simulink model "IEEE14_case"  (R2024b)
settings: Solver=FixedStepAuto  StartTime=0  StopTime=2  FixedStep=1e-7  RelTol=1e-3
values from neighbouring files (symbols this model uses):
  GFL_15_Bva = 0.009    [IEEE14_parameters.m]
  GFL_15_C_bus_pu = 7.179419    [IEEE14_parameters.m]
  GFL_15_f0 = 60    [IEEE14_parameters.m]
  GFL_15_I_id = 691.26967    [IEEE14_parameters.m]
  GFL_15_I_iq = 691.26967    [IEEE14_parameters.m]
  GFL_15_I_od = 45.2207    [IEEE14_parameters.m]
  GFL_15_I_oq = 45.2207    [IEEE14_parameters.m]
  GFL_15_I_pll = 0.78    [IEEE14_parameters.m]
  GFL_15_Kdi = 0.09    [IEEE14_parameters.m]
  GFL_15_Kdo = 0.9    [IEEE14_parameters.m]
  GFL_15_Kqi = 0.09    [IEEE14_parameters.m]
  GFL_15_Kqo = 0.9    [IEEE14_parameters.m]
  GFL_15_Lg_pu = 0.631447    [IEEE14_parameters.m]
  GFL_15_mode = 1    [IEEE14_parameters.m]
  GFL_15_P_id = 3.7166    [IEEE14_parameters.m]
  GFL_15_P_iq = 3.7166    [IEEE14_parameters.m]
  GFL_15_P_od = 0.4798    [IEEE14_parameters.m]
  GFL_15_P_oq = 0.4798    [IEEE14_parameters.m]
  GFL_15_P_pll = 290.42    [IEEE14_parameters.m]
  GFL_15_Qe_ref = 0.2    [IEEE14_parameters.m]
  GFL_15_Rg_pu = 0.024016    [IEEE14_parameters.m]
  GFL_15_Sbase = 1.000000e+4    (= 10000)    [IEEE14_parameters.m]
  GFL_15_Tdi = 0.01    [IEEE14_parameters.m]
  GFL_15_Tdo = 0.2    [IEEE14_parameters.m]
  GFL_15_Tqi = 0.01    [IEEE14_parameters.m]
  GFL_15_Tqo = 0.2    [IEEE14_parameters.m]
  GFL_15_Vbase = 380    [IEEE14_parameters.m]
  GFL_15_Vdc_ref = 1.011475    [IEEE14_parameters.m]
  GFL_15_Vdcbase = 700    [IEEE14_parameters.m]
  GFL_15_vq_ref = 0    [IEEE14_parameters.m]
  GFL_16_Bva = 0.002    [IEEE14_parameters.m]
  GFL_16_C_bus_pu = 7.179419    [IEEE14_parameters.m]
  GFL_16_f0 = 60    [IEEE14_parameters.m]
  GFL_16_I_id = 691.26967    [IEEE14_parameters.m]
  GFL_16_I_iq = 691.26967    [IEEE14_parameters.m]
  GFL_16_I_od = 45.2207    [IEEE14_parameters.m]
  GFL_16_I_oq = 45.2207    [IEEE14_parameters.m]
  GFL_16_I_pll = 0.78    [IEEE14_parameters.m]
  GFL_16_Kdi = 0.05    [IEEE14_parameters.m]
  GFL_16_Kdo = 0.5    [IEEE14_parameters.m]
  GFL_16_Kqi = 0.05    [IEEE14_parameters.m]
  GFL_16_Kqo = 0.5    [IEEE14_parameters.m]
  GFL_16_Lg_pu = 0.631447    [IEEE14_parameters.m]
  GFL_16_mode = 1    [IEEE14_parameters.m]
  GFL_16_P_id = 3.7166    [IEEE14_parameters.m]
  GFL_16_P_iq = 3.7166    [IEEE14_parameters.m]
  GFL_16_P_od = 0.4798    [IEEE14_parameters.m]
  GFL_16_P_oq = 0.4798    [IEEE14_parameters.m]
  GFL_16_P_pll = 290.42    [IEEE14_parameters.m]
  GFL_16_Qe_ref = 0.2    [IEEE14_parameters.m]
  GFL_16_Rg_pu = 0.024016    [IEEE14_parameters.m]
  GFL_16_Sbase = 1.000000e+4    (= 10000)    [IEEE14_parameters.m]
  GFL_16_Tdi = 0.01    [IEEE14_parameters.m]
  GFL_16_Tdo = 0.2    [IEEE14_parameters.m]
  GFL_16_Tqi = 0.01    [IEEE14_parameters.m]
  GFL_16_Tqo = 0.2    [IEEE14_parameters.m]
  GFL_16_Vbase = 380    [IEEE14_parameters.m]
  GFL_16_Vdc_ref = 1.01144    [IEEE14_parameters.m]
  GFL_16_Vdcbase = 700    [IEEE14_parameters.m]
  GFL_16_vq_ref = 0    [IEEE14_parameters.m]
  GFL_17_Bva = 0.002    [IEEE14_parameters.m]
  GFL_17_C_bus_pu = 7.179419    [IEEE14_parameters.m]
  GFL_17_f0 = 60    [IEEE14_parameters.m]
  GFL_17_I_id = 691.26967    [IEEE14_parameters.m]
  GFL_17_I_iq = 691.26967    [IEEE14_parameters.m]
  GFL_17_I_od = 45.2207    [IEEE14_parameters.m]
  GFL_17_I_oq = 45.2207    [IEEE14_parameters.m]
  GFL_17_I_pll = 0.78    [IEEE14_parameters.m]
  GFL_17_Kdi = 0.05    [IEEE14_parameters.m]
  GFL_17_Kdo = 0.5    [IEEE14_parameters.m]
  GFL_17_Kqi = 0.05    [IEEE14_parameters.m]
  GFL_17_Kqo = 0.5    [IEEE14_parameters.m]
  GFL_17_Lg_pu = 0.631447    [IEEE14_parameters.m]
  GFL_17_mode = 1    [IEEE14_parameters.m]
  GFL_17_P_id = 3.7166    [IEEE14_parameters.m]
  GFL_17_P_iq = 3.7166    [IEEE14_parameters.m]
  GFL_17_P_od = 0.4798    [IEEE14_parameters.m]
  GFL_17_P_oq = 0.4798    [IEEE14_parameters.m]
  GFL_17_P_pll = 290.42    [IEEE14_parameters.m]
  GFL_17_Qe_ref = 0.2    [IEEE14_parameters.m]
  GFL_17_Rg_pu = 0.024016    [IEEE14_parameters.m]
  GFL_17_Sbase = 1.000000e+4    (= 10000)    [IEEE14_parameters.m]
  GFL_17_Tdi = 0.01    [IEEE14_parameters.m]
  GFL_17_Tdo = 0.2    [IEEE14_parameters.m]
  GFL_17_Tqi = 0.01    [IEEE14_parameters.m]
  GFL_17_Tqo = 0.2    [IEEE14_parameters.m]
  GFL_17_Vbase = 380    [IEEE14_parameters.m]
  GFL_17_Vdc_ref = 1.011632    [IEEE14_parameters.m]
  GFL_17_Vdcbase = 700    [IEEE14_parameters.m]
  GFL_17_vq_ref = 0    [IEEE14_parameters.m]
  GFL_18_Bva = 0.002    [IEEE14_parameters.m]
  GFL_18_C_bus_pu = 7.179419    [IEEE14_parameters.m]
  GFL_18_f0 = 60    [IEEE14_parameters.m]
  GFL_18_I_id = 691.26967    [IEEE14_parameters.m]
  GFL_18_I_iq = 691.26967    [IEEE14_parameters.m]
  GFL_18_I_od = 45.2207    [IEEE14_parameters.m]
  GFL_18_I_oq = 45.2207    [IEEE14_parameters.m]
  GFL_18_I_pll = 0.78    [IEEE14_parameters.m]
  GFL_18_Kdi = 0.05    [IEEE14_parameters.m]
  GFL_18_Kdo = 0.5    [IEEE14_parameters.m]
  GFL_18_Kqi = 0.05    [IEEE14_parameters.m]
  GFL_18_Kqo = 0.5    [IEEE14_parameters.m]
  GFL_18_Lg_pu = 0.631447    [IEEE14_parameters.m]
  GFL_18_mode = 1    [IEEE14_parameters.m]
  GFL_18_P_id = 3.7166    [IEEE14_parameters.m]
  GFL_18_P_iq = 3.7166    [IEEE14_parameters.m]
  GFL_18_P_od = 0.4798    [IEEE14_parameters.m]
  GFL_18_P_oq = 0.4798    [IEEE14_parameters.m]
  GFL_18_P_pll = 290.42    [IEEE14_parameters.m]
  GFL_18_Qe_ref = 0.2    [IEEE14_parameters.m]
  GFL_18_Rg_pu = 0.024016    [IEEE14_parameters.m]
  GFL_18_Sbase = 1.000000e+4    (= 10000)    [IEEE14_parameters.m]
  GFL_18_Tdi = 0.01    [IEEE14_parameters.m]
  GFL_18_Tdo = 0.2    [IEEE14_parameters.m]
  GFL_18_Tqi = 0.01    [IEEE14_parameters.m]
  GFL_18_Tqo = 0.2    [IEEE14_parameters.m]
  GFL_18_Vbase = 380    [IEEE14_parameters.m]
  GFL_18_Vdc_ref = 1.011572    [IEEE14_parameters.m]
  GFL_18_Vdcbase = 700    [IEEE14_parameters.m]
  GFL_18_vq_ref = 0    [IEEE14_parameters.m]
  ... (+180 more)
(part 7 of 25)

== system IEEE14_case/AC_1/d_iq_line_4_9_block ==
  note: d_iq_line_4_9 in case14gfl
      | $699.506853548825\,\mathrm{vq}_{\mathrm{bus},4}-376.991118430775\,\mathrm{id}_{\mathrm{line},4,9}-699.506853548825\,\mathrm{vq}_{\mathrm{bus},9}$
      | Automatically generated on 2025-10-09 21:39:28 .
  State_id_line_4_9_5fb10 : Inport
  State_vq_bus_4_2d444 : Inport  Port=2
  State_vq_bus_9_e7de0 : Inport  Port=3
  Add_39299 : Sum
  Constant_-376.991118430775_3ea59 : Constant  Value=-376.991118430775
  Constant_699.506853548825_37d82 : Constant  Value=699.506853548825
  Constant_699.506853548825_6575b : Constant  Value=699.506853548825
  Product_2ea70 : Product
  Product_57b01 : Product
  Product_cf664 : Product
  Subtract_80e4f : Sum  Inputs=+-
  Blockout_d_iq_line_4_9_8879d : Outport
  wires:
  Constant_-376.991118430775_3ea59/1 -> Product_57b01/1
  Product_cf664/1 -> Add_39299/2
  Product_57b01/1 -> Add_39299/1
  State_id_line_4_9_5fb10/1 -> Product_57b01/2
  Constant_699.506853548825_6575b/1 -> Product_cf664/1
  State_vq_bus_4_2d444/1 -> Product_cf664/2
  Product_2ea70/1 -> Subtract_80e4f/2
  Constant_699.506853548825_37d82/1 -> Product_2ea70/1
  State_vq_bus_9_e7de0/1 -> Product_2ea70/2
  Add_39299/1 -> Subtract_80e4f/1
  Subtract_80e4f/1 -> Blockout_d_iq_line_4_9_8879d/1

== system IEEE14_case/AC_1/d_iq_line_5_6_block ==
  note: d_iq_line_5_6 in case14gfl
      | $1605.01907859506\,\mathrm{vq}_{\mathrm{bus},5}-376.991118430775\,\mathrm{id}_{\mathrm{line},5,6}-1605.01907859506\,\mathrm{vq}_{\mathrm{bus},6}$
      | Automatically generated on 2025-10-09 21:39:30 .
  State_id_line_5_6_8d92b : Inport
  State_vq_bus_5_491c0 : Inport  Port=2
  State_vq_bus_6_39104 : Inport  Port=3
  Add_7c3b3 : Sum
  Constant_-376.991118430775_fdd64 : Constant  Value=-376.991118430775
  Constant_1605.01907859506_0c9f5 : Constant  Value=1605.01907859506
  Constant_1605.01907859506_7f4c8 : Constant  Value=1605.01907859506
  Product_35d69 : Product
  Product_b6bdb : Product
  Product_ff1a8 : Product
  Subtract_873d9 : Sum  Inputs=+-
  Blockout_d_iq_line_5_6_9d95c : Outport
  wires:
  Constant_-376.991118430775_fdd64/1 -> Product_ff1a8/1
  Product_ff1a8/1 -> Add_7c3b3/1
  State_id_line_5_6_8d92b/1 -> Product_ff1a8/2
  Constant_1605.01907859506_0c9f5/1 -> Product_35d69/1
  State_vq_bus_5_491c0/1 -> Product_35d69/2
  Product_35d69/1 -> Add_7c3b3/2
  State_vq_bus_6_39104/1 -> Product_b6bdb/2
  Product_b6bdb/1 -> Subtract_873d9/2
  Constant_1605.01907859506_7f4c8/1 -> Product_b6bdb/1
  Add_7c3b3/1 -> Subtract_873d9/1
  Subtract_873d9/1 -> Blockout_d_iq_line_5_6_9d95c/1

== system IEEE14_case/AC_1/d_iq_line_6_11_block ==
  note: d_iq_line_6_11 in case14gfl
      | $1895.38018316126\,\mathrm{vq}_{\mathrm{bus},6}-180.023209796657\,\mathrm{iq}_{\mathrm{line},6,11}-376.991118430775\,\mathrm{id}_{\mathrm{line},6,11}-1895.38018316126\,\mathrm{vq}_{\mathrm{bus},11}$
      | Automatically generated on 2025-10-09 21:39:32 .
  State_id_line_6_11_3e498 : Inport
  State_iq_line_6_11_23688 : Inport  Port=2
  State_vq_bus_11_5a0e6 : Inport  Port=3
  State_vq_bus_6_fa1ab : Inport  Port=4
  Add_f0066 : Sum
  Constant_-376.991118430775_7fe8b : Constant  Value=-376.991118430775
  Constant_180.023209796657_42678 : Constant  Value=180.023209796657
  Constant_1895.38018316126_7900e : Constant  Value=1895.38018316126
  Constant_1895.38018316126_a1828 : Constant  Value=1895.38018316126
  Product_3a14e : Product
  Product_60b79 : Product
  Product_843e4 : Product
  Product_bb537 : Product
  Subtract_7b150 : Sum  Inputs=+-
  Subtract_c1d87 : Sum  Inputs=+-
  Blockout_d_iq_line_6_11_ea354 : Outport
  wires:
  Product_60b79/1 -> Subtract_7b150/1
  Constant_-376.991118430775_7fe8b/1 -> Product_60b79/1
  State_id_line_6_11_3e498/1 -> Product_60b79/2
  Constant_180.023209796657_42678/1 -> Product_3a14e/1
  Product_3a14e/1 -> Subtract_7b150/2
  State_iq_line_6_11_23688/1 -> Product_3a14e/2
  Product_bb537/1 -> Subtract_c1d87/2
  Subtract_7b150/1 -> Subtract_c1d87/1
  Constant_1895.38018316126_a1828/1 -> Product_bb537/1
  State_vq_bus_11_5a0e6/1 -> Product_bb537/2
  Product_843e4/1 -> Add_f0066/2
  Constant_1895.38018316126_7900e/1 -> Product_843e4/1
  State_vq_bus_6_fa1ab/1 -> Product_843e4/2
  Subtract_c1d87/1 -> Add_f0066/1
  Add_f0066/1 -> Blockout_d_iq_line_6_11_ea354/1

== system IEEE14_case/AC_1/d_iq_line_6_12_block ==
  note: d_iq_line_6_12 in case14gfl
      | $1473.7153294663\,\mathrm{vq}_{\mathrm{bus},6}-181.134351144703\,\mathrm{iq}_{\mathrm{line},6,12}-376.991118430775\,\mathrm{id}_{\mathrm{line},6,12}-1473.7153294663\,\mathrm{vq}_{\mathrm{bus},12}$
      | Automatically generated on 2025-10-09 21:39:34 .
  State_id_line_6_12_268a8 : Inport
  State_iq_line_6_12_950d7 : Inport  Port=2
  State_vq_bus_12_69550 : Inport  Port=3
  State_vq_bus_6_e763a : Inport  Port=4
  Add_b7468 : Sum
  Constant_-376.991118430775_f1d4f : Constant  Value=-376.991118430775
  Constant_1473.7153294663_049d6 : Constant  Value=1473.7153294663
  Constant_1473.7153294663_ac463 : Constant  Value=1473.7153294663
  Constant_181.134351144703_38039 : Constant  Value=181.134351144703
  Product_43b5c : Product
  Product_574f5 : Product
  Product_5ec2e : Product
  Product_93b39 : Product
  Subtract_6d476 : Sum  Inputs=+-
  Subtract_ac6c5 : Sum  Inputs=+-
  Blockout_d_iq_line_6_12_bda61 : Outport
  wires:
  Subtract_ac6c5/1 -> Subtract_6d476/1
  Constant_-376.991118430775_f1d4f/1 -> Product_574f5/1
  Product_574f5/1 -> Subtract_ac6c5/1
  State_id_line_6_12_268a8/1 -> Product_574f5/2
  Constant_181.134351144703_38039/1 -> Product_43b5c/1
  Product_43b5c/1 -> Subtract_ac6c5/2
  Product_93b39/1 -> Subtract_6d476/2
  Constant_1473.7153294663_049d6/1 -> Product_93b39/1
  State_iq_line_6_12_950d7/1 -> Product_43b5c/2
  State_vq_bus_12_69550/1 -> Product_93b39/2
  Constant_1473.7153294663_ac463/1 -> Product_5ec2e/1
  State_vq_bus_6_e763a/1 -> Product_5ec2e/2
  Subtract_6d476/1 -> Add_b7468/1
  Product_5ec2e/1 -> Add_b7468/2
  Add_b7468/1 -> Blockout_d_iq_line_6_12_bda61/1

== system IEEE14_case/AC_1/d_iq_line_6_13_block ==
  note: d_iq_line_6_13 in case14gfl
      | $2893.92122845456\,\mathrm{vq}_{\mathrm{bus},6}-191.432889262269\,\mathrm{iq}_{\mathrm{line},6,13}-376.991118430775\,\mathrm{id}_{\mathrm{line},6,13}-2893.92122845456\,\mathrm{vq}_{\mathrm{bus},13}$
      | Automatically generated on 2025-10-09 21:39:36 .
  State_id_line_6_13_f1d85 : Inport
  State_iq_line_6_13_f7b4b : Inport  Port=2
  State_vq_bus_13_5730a : Inport  Port=3
  State_vq_bus_6_f0e31 : Inport  Port=4
  Add_1c903 : Sum
  Constant_-376.991118430775_5ef0e : Constant  Value=-376.991118430775
  Constant_191.432889262269_5c0fd : Constant  Value=191.432889262269
  Constant_2893.92122845456_a0aba : Constant  Value=2893.92122845456
  Constant_2893.92122845456_a4a61 : Constant  Value=2893.92122845456
  Product_0336c : Product
  Product_1b8db : Product
  Product_302cd : Product
  Product_77864 : Product
  Subtract_80e31 : Sum  Inputs=+-
  Subtract_b1026 : Sum  Inputs=+-
  Blockout_d_iq_line_6_13_6bd96 : Outport
  wires:
  Constant_-376.991118430775_5ef0e/1 -> Product_0336c/1
  Constant_191.432889262269_5c0fd/1 -> Product_1b8db/1
  State_id_line_6_13_f1d85/1 -> Product_0336c/2
  Product_1b8db/1 -> Subtract_b1026/2
  State_iq_line_6_13_f7b4b/1 -> Product_1b8db/2
  Product_77864/1 -> Subtract_80e31/2
  Constant_2893.92122845456_a0aba/1 -> Product_77864/1
  Product_0336c/1 -> Subtract_b1026/1
  State_vq_bus_13_5730a/1 -> Product_77864/2
  Subtract_b1026/1 -> Subtract_80e31/1
  Product_302cd/1 -> Add_1c903/2
  Constant_2893.92122845456_a4a61/1 -> Product_302cd/1
  State_vq_bus_6_f0e31/1 -> Product_302cd/2
  Subtract_80e31/1 -> Add_1c903/1
  Add_1c903/1 -> Blockout_d_iq_line_6_13_6bd96/1

== system IEEE14_case/AC_1/d_iq_line_7_8_block ==
  note: d_iq_line_7_8 in case14gfl
      | $2140.17098172453\,\mathrm{vq}_{\mathrm{bus},7}-376.991118430775\,\mathrm{id}_{\mathrm{line},7,8}-2140.17098172453\,\mathrm{vq}_{\mathrm{bus},8}$
      | Automatically generated on 2025-10-09 21:39:38 .
  State_id_line_7_8_32461 : Inport
  State_vq_bus_7_4632e : Inport  Port=2
  State_vq_bus_8_957c7 : Inport  Port=3
  Add_fd8d6 : Sum
  Constant_-376.991118430775_d615e : Constant  Value=-376.991118430775
  Constant_2140.17098172453_9f9e4 : Constant  Value=2140.17098172453
  Constant_2140.17098172453_c3816 : Constant  Value=2140.17098172453
  Product_142e7 : Product
  Product_f2e78 : Product
  Product_f7504 : Product
  Subtract_6e91e : Sum  Inputs=+-
  Blockout_d_iq_line_7_8_a0a04 : Outport
  wires:
  Constant_-376.991118430775_d615e/1 -> Product_f2e78/1
  Product_f2e78/1 -> Add_fd8d6/1
  State_id_line_7_8_32461/1 -> Product_f2e78/2
  Constant_2140.17098172453_c3816/1 -> Product_142e7/1
  Product_142e7/1 -> Add_fd8d6/2
  Product_f7504/1 -> Subtract_6e91e/2
  Constant_2140.17098172453_9f9e4/1 -> Product_f7504/1
  State_vq_bus_7_4632e/1 -> Product_142e7/2
  State_vq_bus_8_957c7/1 -> Product_f7504/2
  Add_fd8d6/1 -> Subtract_6e91e/1
  Subtract_6e91e/1 -> Blockout_d_iq_line_7_8_a0a04/1

== system IEEE14_case/AC_1/d_iq_line_7_9_block ==
  note: d_iq_line_7_9 in case14gfl
      | $3426.88045114785\,\mathrm{vq}_{\mathrm{bus},7}-376.991118430775\,\mathrm{id}_{\mathrm{line},7,9}-3426.88045114785\,\mathrm{vq}_{\mathrm{bus},9}$
      | Automatically generated on 2025-10-09 21:39:40 .
  State_id_line_7_9_a5037 : Inport
  State_vq_bus_7_de92f : Inport  Port=2
  State_vq_bus_9_3c7a5 : Inport  Port=3
  Add_30ef7 : Sum
  Constant_-376.991118430775_e9a53 : Constant  Value=-376.991118430775
  Constant_3426.88045114785_151c5 : Constant  Value=3426.88045114785
  Constant_3426.88045114785_ad75e : Constant  Value=3426.88045114785
  Product_648d8 : Product
  Product_dc9ab : Product
  Product_e3dd0 : Product
  Subtract_73145 : Sum  Inputs=+-
  Blockout_d_iq_line_7_9_01bdc : Outport
  wires:
  State_vq_bus_9_3c7a5/1 -> Product_dc9ab/2
  Constant_-376.991118430775_e9a53/1 -> Product_e3dd0/1
  Product_dc9ab/1 -> Subtract_73145/2
  Product_e3dd0/1 -> Add_30ef7/1
  Constant_3426.88045114785_151c5/1 -> Product_dc9ab/1
  State_id_line_7_9_a5037/1 -> Product_e3dd0/2
  Constant_3426.88045114785_ad75e/1 -> Product_648d8/1
  State_vq_bus_7_de92f/1 -> Product_648d8/2
  Product_648d8/1 -> Add_30ef7/2
  Add_30ef7/1 -> Subtract_73145/1
  Subtract_73145/1 -> Blockout_d_iq_line_7_9_01bdc/1

== system IEEE14_case/AC_1/d_iq_line_9_10_block ==
  note: d_iq_line_9_10 in case14gfl
      | $4461.43335421036\,\mathrm{vq}_{\mathrm{bus},9}-141.918194997431\,\mathrm{iq}_{\mathrm{line},9,10}-376.991118430775\,\mathrm{id}_{\mathrm{line},9,10}-4461.43335421036\,\mathrm{vq}_{\mathrm{bus},10}$
      | Automatically generated on 2025-10-09 21:39:42 .
  State_id_line_9_10_7d192 : Inport
  State_iq_line_9_10_78cd2 : Inport  Port=2
  State_vq_bus_10_aebb4 : Inport  Port=3
  State_vq_bus_9_d6463 : Inport  Port=4
  Add_9c341 : Sum
  Constant_-376.991118430775_01110 : Constant  Value=-376.991118430775
  Constant_141.918194997431_f967c : Constant  Value=141.918194997431
  Constant_4461.43335421036_69f6f : Constant  Value=4461.43335421036
  Constant_4461.43335421036_9672c : Constant  Value=4461.43335421036
  Product_02b9f : Product
  Product_1253c : Product
  Product_45f04 : Product
  Product_d2758 : Product
  Subtract_137d4 : Sum  Inputs=+-
  Subtract_6b3b6 : Sum  Inputs=+-
  Blockout_d_iq_line_9_10_9f0b6 : Outport
  wires:
  Constant_-376.991118430775_01110/1 -> Product_1253c/1
  Add_9c341/1 -> Blockout_d_iq_line_9_10_9f0b6/1
  State_id_line_9_10_7d192/1 -> Product_1253c/2
  Constant_141.918194997431_f967c/1 -> Product_45f04/1
  Product_45f04/1 -> Subtract_137d4/2
  State_vq_bus_10_aebb4/1 -> Product_02b9f/2
  State_iq_line_9_10_78cd2/1 -> Product_45f04/2
  Product_1253c/1 -> Subtract_137d4/1
  Constant_4461.43335421036_69f6f/1 -> Product_02b9f/1
  Subtract_137d4/1 -> Subtract_6b3b6/1
  Product_02b9f/1 -> Subtract_6b3b6/2
  Product_d2758/1 -> Add_9c341/2
  Constant_4461.43335421036_9672c/1 -> Product_d2758/1
  State_vq_bus_9_d6463/1 -> Product_d2758/2
  Subtract_6b3b6/1 -> Add_9c341/1

== system IEEE14_case/AC_1/d_iq_line_9_14_block ==
  note: d_iq_line_9_14 in case14gfl
      | $1394.30105196677\,\mathrm{vq}_{\mathrm{bus},9}-177.229606715496\,\mathrm{iq}_{\mathrm{line},9,14}-376.991118430775\,\mathrm{id}_{\mathrm{line},9,14}-1394.30105196677\,\mathrm{vq}_{\mathrm{bus},14}$
      | Automatically generated on 2025-10-09 21:39:45 .
  State_id_line_9_14_dd4a4 : Inport
  State_iq_line_9_14_07292 : Inport  Port=2
  State_vq_bus_14_753fc : Inport  Port=3
  State_vq_bus_9_d4758 : Inport  Port=4
  Add_8f103 : Sum
  Constant_-376.991118430775_6bc62 : Constant  Value=-376.991118430775
  Constant_1394.30105196677_50c0c : Constant  Value=1394.30105196677
  Constant_1394.30105196677_acb93 : Constant  Value=1394.30105196677
  Constant_177.229606715496_1731d : Constant  Value=177.229606715496
  Product_21531 : Product
  Product_30771 : Product
  Product_33e78 : Product
  Product_cf39f : Product
  Subtract_51c64 : Sum  Inputs=+-
  Subtract_b0fd6 : Sum  Inputs=+-
  Blockout_d_iq_line_9_14_f1895 : Outport
  wires:
  Constant_-376.991118430775_6bc62/1 -> Product_21531/1
  State_id_line_9_14_dd4a4/1 -> Product_21531/2
  Subtract_b0fd6/1 -> Subtract_51c64/1
  Constant_177.229606715496_1731d/1 -> Product_30771/1
  Product_30771/1 -> Subtract_b0fd6/2
  Product_cf39f/1 -> Subtract_51c64/2
  Constant_1394.30105196677_50c0c/1 -> Product_cf39f/1
  State_iq_line_9_14_07292/1 -> Product_30771/2
  Product_21531/1 -> Subtract_b0fd6/1
  State_vq_bus_14_753fc/1 -> Product_cf39f/2
  Product_33e78/1 -> Add_8f103/2
  Constant_1394.30105196677_acb93/1 -> Product_33e78/1
  State_vq_bus_9_d4758/1 -> Product_33e78/2
  Subtract_51c64/1 -> Add_8f103/1
  Add_8f103/1 -> Blockout_d_iq_line_9_14_f1895/1

== system IEEE14_case/AC_1/d_iq_load_10_block ==
  note: d_iq_load_10 in case14gfl
      | $60.6278129379132\,\mathrm{vq}_{\mathrm{bus},10}-584.986218254651\,\mathrm{iq}_{\mathrm{load},10}-376.991118430775\,\mathrm{id}_{\mathrm{load},10}$
      | Automatically generated on 2025-10-09 21:39:02 .
  State_id_load_10_0a094 : Inport
  State_iq_load_10_0f9f7 : Inport  Port=2
  State_vq_bus_10_81f02 : Inport  Port=3
  Add_d132c : Sum
  Constant_-376.991118430775_0f5ea : Constant  Value=-376.991118430775
  Constant_584.986218254651_56ed2 : Constant  Value=584.986218254651
  Constant_60.6278129379132_5da5b : Constant  Value=60.6278129379132
  Product_310ba : Product
  Product_360f0 : Product
  Product_4d8c0 : Product
  Subtract_ea92d : Sum  Inputs=+-
  Blockout_d_iq_load_10_8a684 : Outport
  wires:
  State_id_load_10_0a094/1 -> Product_4d8c0/2
  Constant_-376.991118430775_0f5ea/1 -> Product_4d8c0/1
  Constant_584.986218254651_56ed2/1 -> Product_360f0/1
  Product_360f0/1 -> Subtract_ea92d/2
  Product_310ba/1 -> Add_d132c/2
  Constant_60.6278129379132_5da5b/1 -> Product_310ba/1
  State_iq_load_10_0f9f7/1 -> Product_360f0/2
  Product_4d8c0/1 -> Subtract_ea92d/1
  State_vq_bus_10_81f02/1 -> Product_310ba/2
  Subtract_ea92d/1 -> Add_d132c/1
  Add_d132c/1 -> Blockout_d_iq_load_10_8a684/1

== system IEEE14_case/AC_1/d_iq_load_11_block ==
  note: d_iq_load_11 in case14gfl
      | $26.9582940185634\,\mathrm{vq}_{\mathrm{bus},11}-733.038285837618\,\mathrm{iq}_{\mathrm{load},11}-376.991118430775\,\mathrm{id}_{\mathrm{load},11}$
      | Automatically generated on 2025-10-09 21:39:04 .
  State_id_load_11_9ab2f : Inport
  State_iq_load_11_f52d6 : Inport  Port=2
  State_vq_bus_11_ff375 : Inport  Port=3
  Add_de68f : Sum
  Constant_-376.991118430775_db176 : Constant  Value=-376.991118430775
  Constant_26.9582940185634_925bd : Constant  Value=26.9582940185634
  Constant_733.038285837618_6ff3b : Constant  Value=733.038285837618
  Product_491fa : Product
  Product_5b80d : Product
  Product_c6838 : Product
  Subtract_79916 : Sum  Inputs=+-
  Blockout_d_iq_load_11_90745 : Outport
  wires:
  Constant_-376.991118430775_db176/1 -> Product_491fa/1
  Constant_733.038285837618_6ff3b/1 -> Product_c6838/1
  Product_c6838/1 -> Subtract_79916/2
  State_id_load_11_9ab2f/1 -> Product_491fa/2
  State_iq_load_11_f52d6/1 -> Product_c6838/2
  Product_491fa/1 -> Subtract_79916/1
  State_vq_bus_11_ff375/1 -> Product_5b80d/2
  Product_5b80d/1 -> Add_de68f/2
  Constant_26.9582940185634_925bd/1 -> Product_5b80d/1
  Subtract_79916/1 -> Add_de68f/1
  Add_de68f/1 -> Blockout_d_iq_load_11_90745/1

== system IEEE14_case/AC_1/d_iq_load_12_block ==
  note: d_iq_load_12 in case14gfl
      | $77.623450441014\,\mathrm{vq}_{\mathrm{bus},12}-1437.27863901733\,\mathrm{iq}_{\mathrm{load},12}-376.991118430775\,\mathrm{id}_{\mathrm{load},12}$
      | Automatically generated on 2025-10-09 21:39:06 .
  State_id_load_12_0975f : Inport
  State_iq_load_12_acbdc : Inport  Port=2
  State_vq_bus_12_83802 : Inport  Port=3
  Add_36107 : Sum
  Constant_-376.991118430775_9dcd8 : Constant  Value=-376.991118430775
  Constant_1437.27863901733_57e09 : Constant  Value=1437.27863901733
  Constant_77.623450441014_2708c : Constant  Value=77.623450441014
  Product_a0656 : Product
  Product_c6599 : Product
  Product_e67ca : Product
  Subtract_88912 : Sum  Inputs=+-
  Blockout_d_iq_load_12_9f109 : Outport
  wires:
  State_id_load_12_0975f/1 -> Product_c6599/2
  Constant_-376.991118430775_9dcd8/1 -> Product_c6599/1
  Constant_1437.27863901733_57e09/1 -> Product_e67ca/1
  Product_e67ca/1 -> Subtract_88912/2
  Product_a0656/1 -> Add_36107/2
  Constant_77.623450441014_2708c/1 -> Product_a0656/1
  State_iq_load_12_acbdc/1 -> Product_e67ca/2
  Product_c6599/1 -> Subtract_88912/1
  State_vq_bus_12_83802/1 -> Product_a0656/2
  Subtract_88912/1 -> Add_36107/1
  Add_36107/1 -> Blockout_d_iq_load_12_9f109/1

== system IEEE14_case/AC_1/d_iq_load_13_block ==
  note: d_iq_load_13 in case14gfl
      | $118.242352238424\,\mathrm{vq}_{\mathrm{bus},13}-877.479327381977\,\mathrm{iq}_{\mathrm{load},13}-376.991118430775\,\mathrm{id}_{\mathrm{load},13}$
      | Automatically generated on 2025-10-09 21:39:07 .
  State_id_load_13_29b8c : Inport
  State_iq_load_13_dc329 : Inport  Port=2
  State_vq_bus_13_7eda7 : Inport  Port=3
  Add_196d0 : Sum
  Constant_-376.991118430775_54985 : Constant  Value=-376.991118430775
  Constant_118.242352238424_0be43 : Constant  Value=118.242352238424
  Constant_877.479327381977_663e1 : Constant  Value=877.479327381977
  Product_31344 : Product
  Product_8bd14 : Product
  Product_fe9c5 : Product
  Subtract_4cd3e : Sum  Inputs=+-
  Blockout_d_iq_load_13_714c3 : Outport
  wires:
  Constant_-376.991118430775_54985/1 -> Product_8bd14/1
  Constant_877.479327381977_663e1/1 -> Product_fe9c5/1
  Product_fe9c5/1 -> Subtract_4cd3e/2
  State_id_load_13_29b8c/1 -> Product_8bd14/2
  State_iq_load_13_dc329/1 -> Product_fe9c5/2
  Product_8bd14/1 -> Subtract_4cd3e/1
  State_vq_bus_13_7eda7/1 -> Product_31344/2
  Product_31344/1 -> Add_196d0/2
  Constant_118.242352238424_0be43/1 -> Product_31344/1
  Subtract_4cd3e/1 -> Add_196d0/1
  Add_196d0/1 -> Blockout_d_iq_load_13_714c3/1

== system IEEE14_case/AC_1/d_iq_load_14_block ==
  note: d_iq_load_14 in case14gfl
      | $156.099712947555\,\mathrm{vq}_{\mathrm{bus},14}-1123.43353292371\,\mathrm{iq}_{\mathrm{load},14}-376.991118430775\,\mathrm{id}_{\mathrm{load},14}$
      | Automatically generated on 2025-10-09 21:39:10 .
  State_id_load_14_07147 : Inport
  State_iq_load_14_ef373 : Inport  Port=2
  State_vq_bus_14_cd634 : Inport  Port=3
  Add_ad506 : Sum
  Constant_-376.991118430775_2060a : Constant  Value=-376.991118430775
  Constant_1123.43353292371_be503 : Constant  Value=1123.43353292371
  Constant_156.099712947555_a0693 : Constant  Value=156.099712947555
  Product_1a567 : Product
  Product_350ab : Product
  Product_37ef4 : Product
  Subtract_77877 : Sum  Inputs=+-
  Blockout_d_iq_load_14_aff57 : Outport
  wires:
  Constant_-376.991118430775_2060a/1 -> Product_350ab/1
  State_id_load_14_07147/1 -> Product_350ab/2
  Constant_1123.43353292371_be503/1 -> Product_1a567/1
  Product_1a567/1 -> Subtract_77877/2
  State_iq_load_14_ef373/1 -> Product_1a567/2
  Product_350ab/1 -> Subtract_77877/1
  State_vq_bus_14_cd634/1 -> Product_37ef4/2
  Add_ad506/1 -> Blockout_d_iq_load_14_aff57/1
  Product_37ef4/1 -> Add_ad506/2
  Constant_156.099712947555_a0693/1 -> Product_37ef4/1
  Subtract_77877/1 -> Add_ad506/1

== system IEEE14_case/AC_1/d_iq_load_2_block ==
  note: d_iq_load_2 in case14gfl
      | $171.84447318187\,\mathrm{vq}_{\mathrm{bus},2}-644.150178736049\,\mathrm{iq}_{\mathrm{load},2}-376.991118430775\,\mathrm{id}_{\mathrm{load},2}$
      | Automatically generated on 2025-10-09 21:38:51 .
  State_id_load_2_e4c0e : Inport
  State_iq_load_2_39818 : Inport  Port=2
  State_vq_bus_2_25b3a : Inport  Port=3
  Add_3d549 : Sum
  Constant_-376.991118430775_94e96 : Constant  Value=-376.991118430775
  Constant_171.84447318187_7b304 : Constant  Value=171.84447318187
  Constant_644.150178736049_dd5b8 : Constant  Value=644.150178736049
  Product_4ba83 : Product
  Product_91cb5 : Product
  Product_b6ea5 : Product
  Subtract_dfcdb : Sum  Inputs=+-
  Blockout_d_iq_load_2_9dea5 : Outport
  wires:
  Constant_-376.991118430775_94e96/1 -> Product_4ba83/1
  State_id_load_2_e4c0e/1 -> Product_4ba83/2
  Constant_644.150178736049_dd5b8/1 -> Product_b6ea5/1
  Product_b6ea5/1 -> Subtract_dfcdb/2
  State_iq_load_2_39818/1 -> Product_b6ea5/2
  Product_4ba83/1 -> Subtract_dfcdb/1
  State_vq_bus_2_25b3a/1 -> Product_91cb5/2
  Product_91cb5/1 -> Add_3d549/2
  Constant_171.84447318187_7b304/1 -> Product_91cb5/1
  Subtract_dfcdb/1 -> Add_3d549/1
  Add_3d549/1 -> Blockout_d_iq_load_2_9dea5/1

== system IEEE14_case/AC_1/d_iq_load_3_block ==
  note: d_iq_load_3 in case14gfl
      | $1796.20019807427\,\mathrm{vq}_{\mathrm{bus},3}-1869.08228190416\,\mathrm{iq}_{\mathrm{load},3}-376.991118430775\,\mathrm{id}_{\mathrm{load},3}$
      | Automatically generated on 2025-10-09 21:38:53 .
  State_id_load_3_d79a9 : Inport
  State_iq_load_3_276a1 : Inport  Port=2
  State_vq_bus_3_60dd0 : Inport  Port=3
  Add_0c614 : Sum
  Constant_-376.991118430775_2482b : Constant  Value=-376.991118430775
  Constant_1796.20019807427_a8905 : Constant  Value=1796.20019807427
  Constant_1869.08228190416_d8dae : Constant  Value=1869.08228190416
  Product_0f39e : Product
  Product_a564c : Product
  Product_a7995 : Product
  Subtract_ed118 : Sum  Inputs=+-
  Blockout_d_iq_load_3_49ef1 : Outport
  wires:
  Constant_-376.991118430775_2482b/1 -> Product_a564c/1
  State_id_load_3_d79a9/1 -> Product_a564c/2
  Constant_1869.08228190416_d8dae/1 -> Product_0f39e/1
  Product_0f39e/1 -> Subtract_ed118/2
  Product_a7995/1 -> Add_0c614/2
  Constant_1796.20019807427_a8905/1 -> Product_a7995/1
  State_iq_load_3_276a1/1 -> Product_0f39e/2
  Product_a564c/1 -> Subtract_ed118/1
  State_vq_bus_3_60dd0/1 -> Product_a7995/2
  Subtract_ed118/1 -> Add_0c614/1
  Add_0c614/1 -> Blockout_d_iq_load_3_49ef1/1

== system IEEE14_case/AC_1/d_iq_load_4_block ==
  note: d_iq_load_4 in case14gfl
      | $2007.66181460144\,\mathrm{vq}_{\mathrm{bus},4}-4620.55781051053\,\mathrm{iq}_{\mathrm{load},4}-376.991118430775\,\mathrm{id}_{\mathrm{load},4}$
      | Automatically generated on 2025-10-09 21:38:54 .
  State_id_load_4_3f12c : Inport
  State_iq_load_4_d8cb8 : Inport  Port=2
  State_vq_bus_4_a0870 : Inport  Port=3
  Add_0450e : Sum
  Constant_-376.991118430775_4db17 : Constant  Value=-376.991118430775
  Constant_2007.66181460144_721d3 : Constant  Value=2007.66181460144
  Constant_4620.55781051053_0d5fe : Constant  Value=4620.55781051053
  Product_5cc4f : Product
  Product_8d04b : Product
  Product_ee59e : Product
  Subtract_4e0cc : Sum  Inputs=+-
  Blockout_d_iq_load_4_a1a6f : Outport
  wires:
  Constant_-376.991118430775_4db17/1 -> Product_5cc4f/1
  Constant_4620.55781051053_0d5fe/1 -> Product_ee59e/1
  Product_ee59e/1 -> Subtract_4e0cc/2
  State_id_load_4_3f12c/1 -> Product_5cc4f/2
  State_iq_load_4_d8cb8/1 -> Product_ee59e/2
  Product_8d04b/1 -> Add_0450e/2
  Constant_2007.66181460144_721d3/1 -> Product_8d04b/1
  Product_5cc4f/1 -> Subtract_4e0cc/1
  State_vq_bus_4_a0870/1 -> Product_8d04b/2
  Subtract_4e0cc/1 -> Add_0450e/1
  Add_0450e/1 -> Blockout_d_iq_load_4_a1a6f/1

== system IEEE14_case/AC_1/d_iq_load_5_block ==
  note: d_iq_load_5 in case14gfl
      | $126.842875202809\,\mathrm{vq}_{\mathrm{bus},5}-1790.70781254618\,\mathrm{iq}_{\mathrm{load},5}-376.991118430775\,\mathrm{id}_{\mathrm{load},5}$
      | Automatically generated on 2025-10-09 21:38:56 .
  State_id_load_5_e43f2 : Inport
  State_iq_load_5_ed9b4 : Inport  Port=2
  State_vq_bus_5_cfb62 : Inport  Port=3
  Add_95bc5 : Sum
  Constant_-376.991118430775_cfec7 : Constant  Value=-376.991118430775
  Constant_126.842875202809_9c550 : Constant  Value=126.842875202809
  Constant_1790.70781254618_74583 : Constant  Value=1790.70781254618
  Product_15d6e : Product
  Product_20eec : Product
  Product_b8d9d : Product
  Subtract_fe7d7 : Sum  Inputs=+-
  Blockout_d_iq_load_5_ab2ba : Outport
  wires:
  State_id_load_5_e43f2/1 -> Product_20eec/2
  Constant_-376.991118430775_cfec7/1 -> Product_20eec/1
  Constant_1790.70781254618_74583/1 -> Product_15d6e/1
  Product_15d6e/1 -> Subtract_fe7d7/2
  State_iq_load_5_ed9b4/1 -> Product_15d6e/2
  Product_20eec/1 -> Subtract_fe7d7/1
  Product_b8d9d/1 -> Add_95bc5/2
  Constant_126.842875202809_9c550/1 -> Product_b8d9d/1
  State_vq_bus_5_cfb62/1 -> Product_b8d9d/2
  Subtract_fe7d7/1 -> Add_95bc5/1
  Add_95bc5/1 -> Blockout_d_iq_load_5_ab2ba/1

== system IEEE14_case/AC_1/d_iq_load_6_block ==
  note: d_iq_load_6 in case14gfl
      | $79.7688488749381\,\mathrm{vq}_{\mathrm{bus},6}-562.973403523291\,\mathrm{iq}_{\mathrm{load},6}-376.991118430775\,\mathrm{id}_{\mathrm{load},6}$
      | Automatically generated on 2025-10-09 21:38:58 .
  State_id_load_6_8bda4 : Inport
  State_iq_load_6_40498 : Inport  Port=2
  State_vq_bus_6_34215 : Inport  Port=3
  Add_60b3d : Sum
  Constant_-376.991118430775_c5b6b : Constant  Value=-376.991118430775
  Constant_562.973403523291_b5b01 : Constant  Value=562.973403523291
  Constant_79.7688488749381_4dbb0 : Constant  Value=79.7688488749381
  Product_ab997 : Product
  Product_aeba3 : Product
  Product_e7d90 : Product
  Subtract_99f0e : Sum  Inputs=+-
  Blockout_d_iq_load_6_d9bfd : Outport
  wires:
  Constant_-376.991118430775_c5b6b/1 -> Product_aeba3/1
  State_id_load_6_8bda4/1 -> Product_aeba3/2
  Constant_562.973403523291_b5b01/1 -> Product_e7d90/1
  Product_e7d90/1 -> Subtract_99f0e/2
  State_iq_load_6_40498/1 -> Product_e7d90/2
  Product_aeba3/1 -> Subtract_99f0e/1
  State_vq_bus_6_34215/1 -> Product_ab997/2
  Product_ab997/1 -> Add_60b3d/2
  Constant_79.7688488749381_4dbb0/1 -> Product_ab997/1
  Subtract_99f0e/1 -> Add_60b3d/1
  Add_60b3d/1 -> Blockout_d_iq_load_6_d9bfd/1

== system IEEE14_case/AC_1/d_iq_load_9_block ==
  note: d_iq_load_9 in case14gfl
      | $214.658794552347\,\mathrm{vq}_{\mathrm{bus},9}-669.954096006498\,\mathrm{iq}_{\mathrm{load},9}-376.991118430775\,\mathrm{id}_{\mathrm{load},9}$
      | Automatically generated on 2025-10-09 21:39:00 .
  State_id_load_9_c0f8a : Inport
  State_iq_load_9_3e6fb : Inport  Port=2
  State_vq_bus_9_1c480 : Inport  Port=3
  Add_e4dd6 : Sum
  Constant_-376.991118430775_e7f7f : Constant  Value=-376.991118430775
  Constant_214.658794552347_a4e84 : Constant  Value=214.658794552347
  Constant_669.954096006498_74fba : Constant  Value=669.954096006498
  Product_06427 : Product
  Product_4c7f8 : Product
  Product_84118 : Product
  Subtract_6bfbd : Sum  Inputs=+-
  Blockout_d_iq_load_9_c9e01 : Outport
  wires:
  Constant_-376.991118430775_e7f7f/1 -> Product_06427/1
  State_iq_load_9_3e6fb/1 -> Product_84118/2
  State_id_load_9_c0f8a/1 -> Product_06427/2
  Constant_669.954096006498_74fba/1 -> Product_84118/1
  Product_84118/1 -> Subtract_6bfbd/2
  Product_06427/1 -> Subtract_6bfbd/1
  State_vq_bus_9_1c480/1 -> Product_4c7f8/2
  Product_4c7f8/1 -> Add_e4dd6/2
  Constant_214.658794552347_a4e84/1 -> Product_4c7f8/1
  Subtract_6bfbd/1 -> Add_e4dd6/1
  Add_e4dd6/1 -> Blockout_d_iq_load_9_c9e01/1

== system IEEE14_case/AC_1/d_vd_bus_10_block ==
  note: d_vd_bus_10 in case14gfl
      | $1749.67102824962\,\mathrm{id}_{\mathrm{bus},10}+376.991118430775\,\mathrm{vq}_{\mathrm{bus},10}$
      | Automatically generated on 2025-10-09 21:38:36 .
  Alge_id_bus_10_8b36b : Inport
  State_vq_bus_10_6f6de : Inport  Port=2
  Add_a3e5f : Sum
  Constant_1749.67102824962_7c636 : Constant  Value=1749.67102824962
  Constant_376.991118430775_b349f : Constant  Value=376.991118430775
  Product_26821 : Product
  Product_27b5f : Product
  Blockout_d_vd_bus_10_484a7 : Outport
  wires:
  State_vq_bus_10_6f6de/1 -> Product_26821/2
  Constant_1749.67102824962_7c636/1 -> Product_27b5f/1
  Product_26821/1 -> Add_a3e5f/2
  Constant_376.991118430775_b349f/1 -> Product_26821/1
  Alge_id_bus_10_8b36b/1 -> Product_27b5f/2
  Product_27b5f/1 -> Add_a3e5f/1
  Add_a3e5f/1 -> Blockout_d_vd_bus_10_484a7/1

== system IEEE14_case/AC_1/d_vd_bus_11_block ==
  note: d_vd_bus_11 in case14gfl
      | $9002.98797417909\,\mathrm{id}_{\mathrm{bus},11}+376.991118430775\,\mathrm{vq}_{\mathrm{bus},11}$
      | Automatically generated on 2025-10-09 21:38:37 .
  Alge_id_bus_11_fad28 : Inport
  State_vq_bus_11_98fc3 : Inport  Port=2
  Add_c4251 : Sum
  Constant_376.991118430775_68760 : Constant  Value=376.991118430775
  Constant_9002.98797417909_f6ff4 : Constant  Value=9002.98797417909
  Product_61a89 : Product
  Product_8f0d7 : Product
  Blockout_d_vd_bus_11_0b5d5 : Outport
  wires:
  Alge_id_bus_11_fad28/1 -> Product_8f0d7/2
  Constant_9002.98797417909_f6ff4/1 -> Product_8f0d7/1
  Product_61a89/1 -> Add_c4251/2
  Constant_376.991118430775_68760/1 -> Product_61a89/1
  State_vq_bus_11_98fc3/1 -> Product_61a89/2
  Product_8f0d7/1 -> Add_c4251/1
  Add_c4251/1 -> Blockout_d_vd_bus_11_0b5d5/1

== system IEEE14_case/AC_1/d_vd_bus_12_block ==
  note: d_vd_bus_12 in case14gfl
      | $3672.44450708959\,\mathrm{id}_{\mathrm{bus},12}+376.991118430775\,\mathrm{vq}_{\mathrm{bus},12}$
      | Automatically generated on 2025-10-09 21:38:39 .
  Alge_id_bus_12_768d8 : Inport
  State_vq_bus_12_ee0ac : Inport  Port=2
  Add_1268c : Sum
  Constant_3672.44450708959_414e0 : Constant  Value=3672.44450708959
  Constant_376.991118430775_f9b2f : Constant  Value=376.991118430775
  Product_2ec96 : Product
  Product_d4bb7 : Product
  Blockout_d_vd_bus_12_63d51 : Outport
  wires:
  Add_1268c/1 -> Blockout_d_vd_bus_12_63d51/1
  Constant_3672.44450708959_414e0/1 -> Product_d4bb7/1
  Alge_id_bus_12_768d8/1 -> Product_d4bb7/2
  Constant_376.991118430775_f9b2f/1 -> Product_2ec96/1
  Product_d4bb7/1 -> Add_1268c/1
  State_vq_bus_12_ee0ac/1 -> Product_2ec96/2
  Product_2ec96/1 -> Add_1268c/2

== system IEEE14_case/AC_1/d_vd_bus_13_block ==
  note: d_vd_bus_13 in case14gfl
      | $2548.2341972351\,\mathrm{id}_{\mathrm{bus},13}+376.991118430775\,\mathrm{vq}_{\mathrm{bus},13}$
      | Automatically generated on 2025-10-09 21:38:40 .
  Alge_id_bus_13_3078a : Inport
  State_vq_bus_13_424b0 : Inport  Port=2
  Add_3ff77 : Sum
  Constant_2548.2341972351_a6f15 : Constant  Value=2548.2341972351
  Constant_376.991118430775_7edab : Constant  Value=376.991118430775
  Product_471d9 : Product
  Product_5ea4f : Product
  Blockout_d_vd_bus_13_9076d : Outport
  wires:
  Add_3ff77/1 -> Blockout_d_vd_bus_13_9076d/1
  Constant_2548.2341972351_a6f15/1 -> Product_5ea4f/1
  Alge_id_bus_13_3078a/1 -> Product_5ea4f/2
  Product_471d9/1 -> Add_3ff77/2
  Constant_376.991118430775_7edab/1 -> Product_471d9/1
  Product_5ea4f/1 -> Add_3ff77/1
  State_vq_bus_13_424b0/1 -> Product_471d9/2

== system IEEE14_case/AC_1/d_vd_bus_14_block ==
  note: d_vd_bus_14 in case14gfl
      | $20061.7254996805\,\mathrm{id}_{\mathrm{bus},14}+376.991118430775\,\mathrm{vq}_{\mathrm{bus},14}$
      | Automatically generated on 2025-10-09 21:38:42 .
  Alge_id_bus_14_7a3c0 : Inport
  State_vq_bus_14_3a1f7 : Inport  Port=2
  Add_09018 : Sum
  Constant_20061.7254996805_ad767 : Constant  Value=20061.7254996805
  Constant_376.991118430775_38c4b : Constant  Value=376.991118430775
  Product_0d21c : Product
  Product_9c99d : Product
  Blockout_d_vd_bus_14_7c236 : Outport
  wires:
  Constant_20061.7254996805_ad767/1 -> Product_9c99d/1
  Alge_id_bus_14_7a3c0/1 -> Product_9c99d/2
  Product_0d21c/1 -> Add_09018/2
  Constant_376.991118430775_38c4b/1 -> Product_0d21c/1
  Product_9c99d/1 -> Add_09018/1
  State_vq_bus_14_3a1f7/1 -> Product_0d21c/2
  Add_09018/1 -> Blockout_d_vd_bus_14_7c236/1

== system IEEE14_case/AC_1/d_vd_bus_15_block ==
  note: d_vd_bus_15 in case14gfl
      | $37699.1118430775\,\mathrm{id}_{\mathrm{bus},15}+376.991118430775\,\mathrm{vq}_{\mathrm{bus},15}$
      | Automatically generated on 2025-10-09 21:38:43 .
  Alge_id_bus_15_fd09e : Inport
  State_vq_bus_15_3aaea : Inport  Port=2
  Add_0b317 : Sum
  Constant_376.991118430775_00aaa : Constant  Value=376.991118430775
  Constant_37699.1118430775_a5440 : Constant  Value=37699.1118430775
  Product_cad66 : Product
  Product_d5012 : Product
  Blockout_d_vd_bus_15_6b2d1 : Outport
  wires:
  Constant_37699.1118430775_a5440/1 -> Product_cad66/1
  Product_d5012/1 -> Add_0b317/2
  Constant_376.991118430775_00aaa/1 -> Product_d5012/1
  Alge_id_bus_15_fd09e/1 -> Product_cad66/2
  State_vq_bus_15_3aaea/1 -> Product_d5012/2
  Product_cad66/1 -> Add_0b317/1
  Add_0b317/1 -> Blockout_d_vd_bus_15_6b2d1/1

== system IEEE14_case/AC_1/d_vd_bus_16_block ==
  note: d_vd_bus_16 in case14gfl
      | $37699.1118430775\,\mathrm{id}_{\mathrm{bus},16}+376.991118430775\,\mathrm{vq}_{\mathrm{bus},16}$
      | Automatically generated on 2025-10-09 21:38:45 .
  Alge_id_bus_16_8d52e : Inport
  State_vq_bus_16_21a55 : Inport  Port=2
  Add_c7ade : Sum
  Constant_376.991118430775_804af : Constant  Value=376.991118430775
  Constant_37699.1118430775_7bd68 : Constant  Value=37699.1118430775
  Product_435b3 : Product
  Product_53fa4 : Product
  Blockout_d_vd_bus_16_67f66 : Outport
  wires:
  Constant_37699.1118430775_7bd68/1 -> Product_435b3/1
  Product_53fa4/1 -> Add_c7ade/2
  Alge_id_bus_16_8d52e/1 -> Product_435b3/2
  Constant_376.991118430775_804af/1 -> Product_53fa4/1
  State_vq_bus_16_21a55/1 -> Product_53fa4/2
  Product_435b3/1 -> Add_c7ade/1
  Add_c7ade/1 -> Blockout_d_vd_bus_16_67f66/1

== system IEEE14_case/AC_1/d_vd_bus_17_block ==
  note: d_vd_bus_17 in case14gfl
      | $37699.1118430775\,\mathrm{id}_{\mathrm{bus},17}+376.991118430775\,\mathrm{vq}_{\mathrm{bus},17}$
      | Automatically generated on 2025-10-09 21:38:47 .
  Alge_id_bus_17_262b4 : Inport
  State_vq_bus_17_647a1 : Inport  Port=2
  Add_3de89 : Sum
  Constant_376.991118430775_c8c2f : Constant  Value=376.991118430775
  Constant_37699.1118430775_bffe4 : Constant  Value=37699.1118430775
  Product_5c0d6 : Product
  Product_68ad7 : Product
  Blockout_d_vd_bus_17_dc311 : Outport
  wires:
  Add_3de89/1 -> Blockout_d_vd_bus_17_dc311/1
  Constant_37699.1118430775_bffe4/1 -> Product_68ad7/1
  Alge_id_bus_17_262b4/1 -> Product_68ad7/2
  Product_5c0d6/1 -> Add_3de89/2
  Constant_376.991118430775_c8c2f/1 -> Product_5c0d6/1
  Product_68ad7/1 -> Add_3de89/1
  State_vq_bus_17_647a1/1 -> Product_5c0d6/2

== system IEEE14_case/AC_1/d_vd_bus_18_block ==
  note: d_vd_bus_18 in case14gfl
      | $37699.1118430775\,\mathrm{id}_{\mathrm{bus},18}+376.991118430775\,\mathrm{vq}_{\mathrm{bus},18}$
      | Automatically generated on 2025-10-09 21:38:48 .
  Alge_id_bus_18_48e95 : Inport
  State_vq_bus_18_c75a6 : Inport  Port=2
  Add_27cba : Sum
  Constant_376.991118430775_127bc : Constant  Value=376.991118430775
  Constant_37699.1118430775_f9a28 : Constant  Value=37699.1118430775
  Product_322c1 : Product
  Product_5453a : Product
  Blockout_d_vd_bus_18_49967 : Outport
  wires:
  Constant_37699.1118430775_f9a28/1 -> Product_5453a/1
  Alge_id_bus_18_48e95/1 -> Product_5453a/2
  Product_322c1/1 -> Add_27cba/2
  Constant_376.991118430775_127bc/1 -> Product_322c1/1
  Product_5453a/1 -> Add_27cba/1
  State_vq_bus_18_c75a6/1 -> Product_322c1/2
  Add_27cba/1 -> Blockout_d_vd_bus_18_49967/1

== system IEEE14_case/AC_1/d_vd_bus_1_block ==
  note: d_vd_bus_1 in case14gfl
      | $7391.98271432892\,\mathrm{id}_{\mathrm{bus},1}+376.991118430775\,\mathrm{vq}_{\mathrm{bus},1}$
      | Automatically generated on 2025-10-09 21:38:23 .
  Alge_id_bus_1_90b3c : Inport
  State_vq_bus_1_8d526 : Inport  Port=2
  Add_1c0b8 : Sum
  Constant_376.991118430775_8c1e4 : Constant  Value=376.991118430775
  Constant_7391.98271432892_c2a8f : Constant  Value=7391.98271432892
  Product_57029 : Product
  Product_6660f : Product
  Blockout_d_vd_bus_1_52715 : Outport
  wires:
  Constant_7391.98271432892_c2a8f/1 -> Product_57029/1
  Alge_id_bus_1_90b3c/1 -> Product_57029/2
  Product_6660f/1 -> Add_1c0b8/2
  Constant_376.991118430775_8c1e4/1 -> Product_6660f/1
  State_vq_bus_1_8d526/1 -> Product_6660f/2
  Add_1c0b8/1 -> Blockout_d_vd_bus_1_52715/1
  Product_57029/1 -> Add_1c0b8/1

== system IEEE14_case/AC_1/d_vd_bus_2_block ==
  note: d_vd_bus_2 in case14gfl
      | $4564.05712385926\,\mathrm{id}_{\mathrm{bus},2}+376.991118430775\,\mathrm{vq}_{\mathrm{bus},2}$
      | Automatically generated on 2025-10-09 21:38:24 .
  Alge_id_bus_2_b20cd : Inport
  State_vq_bus_2_bcae6 : Inport  Port=2
  Add_71e21 : Sum
  Constant_376.991118430775_c9454 : Constant  Value=376.991118430775
  Constant_4564.05712385926_b3c45 : Constant  Value=4564.05712385926
  Product_65c83 : Product
  Product_7d359 : Product
  Blockout_d_vd_bus_2_7ca8e : Outport
  wires:
  Constant_4564.05712385926_b3c45/1 -> Product_65c83/1
  Alge_id_bus_2_b20cd/1 -> Product_65c83/2
  Product_7d359/1 -> Add_71e21/2
  Constant_376.991118430775_c9454/1 -> Product_7d359/1
  Product_65c83/1 -> Add_71e21/1
  State_vq_bus_2_bcae6/1 -> Product_7d359/2
  Add_71e21/1 -> Blockout_d_vd_bus_2_7ca8e/1

== system IEEE14_case/AC_1/d_vd_bus_3_block ==
  note: d_vd_bus_3 in case14gfl
      | $13321.2409339497\,\mathrm{id}_{\mathrm{bus},3}+376.991118430775\,\mathrm{vq}_{\mathrm{bus},3}$
      | Automatically generated on 2025-10-09 21:38:26 .
  Alge_id_bus_3_b82db : Inport
  State_vq_bus_3_fe7bf : Inport  Port=2
  Add_0338a : Sum
  Constant_13321.2409339497_512f8 : Constant  Value=13321.2409339497
  Constant_376.991118430775_f70c2 : Constant  Value=376.991118430775
  Product_92891 : Product
  Product_ee890 : Product
  Blockout_d_vd_bus_3_5883d : Outport
  wires:
  Add_0338a/1 -> Blockout_d_vd_bus_3_5883d/1
  Constant_13321.2409339497_512f8/1 -> Product_92891/1
  Alge_id_bus_3_b82db/1 -> Product_92891/2
  Product_ee890/1 -> Add_0338a/2
  Constant_376.991118430775_f70c2/1 -> Product_ee890/1
  Product_92891/1 -> Add_0338a/1
  State_vq_bus_3_fe7bf/1 -> Product_ee890/2

== system IEEE14_case/AC_1/d_vd_bus_4_block ==
  note: d_vd_bus_4 in case14gfl
      | $2583.02077551357\,\mathrm{id}_{\mathrm{bus},4}+376.991118430775\,\mathrm{vq}_{\mathrm{bus},4}$
      | Automatically generated on 2025-10-09 21:38:27 .
  Alge_id_bus_4_f94e7 : Inport
  State_vq_bus_4_a1d9b : Inport  Port=2
  Add_04297 : Sum
  Constant_2583.02077551357_562d1 : Constant  Value=2583.02077551357
  Constant_376.991118430775_25894 : Constant  Value=376.991118430775
  Product_bf91e : Product
  Product_eba07 : Product
  Blockout_d_vd_bus_4_c11bd : Outport
  wires:
  Constant_2583.02077551357_562d1/1 -> Product_bf91e/1
  Alge_id_bus_4_f94e7/1 -> Product_bf91e/2
  Constant_376.991118430775_25894/1 -> Product_eba07/1
  Product_eba07/1 -> Add_04297/2
  State_vq_bus_4_a1d9b/1 -> Product_eba07/2
  Product_bf91e/1 -> Add_04297/1
  Add_04297/1 -> Blockout_d_vd_bus_4_c11bd/1

== system IEEE14_case/AC_1/d_vd_bus_5_block ==
  note: d_vd_bus_5 in case14gfl
      | $1402.86696243716\,\mathrm{id}_{\mathrm{bus},5}+376.991118430775\,\mathrm{vq}_{\mathrm{bus},5}$
      | Automatically generated on 2025-10-09 21:38:29 .
  Alge_id_bus_5_3a39c : Inport
  State_vq_bus_5_bfac5 : Inport  Port=2
  Add_800e2 : Sum
  Constant_1402.86696243716_2fe9f : Constant  Value=1402.86696243716
  Constant_376.991118430775_3c04e : Constant  Value=376.991118430775
  Product_db852 : Product
  Product_fcb25 : Product
  Blockout_d_vd_bus_5_c33ea : Outport
  wires:
  Constant_1402.86696243716_2fe9f/1 -> Product_db852/1
  Product_fcb25/1 -> Add_800e2/2
  Constant_376.991118430775_3c04e/1 -> Product_fcb25/1
  Alge_id_bus_5_3a39c/1 -> Product_db852/2
  State_vq_bus_5_bfac5/1 -> Product_fcb25/2
  Product_db852/1 -> Add_800e2/1
  Add_800e2/1 -> Blockout_d_vd_bus_5_c33ea/1

== system IEEE14_case/AC_1/d_vd_bus_6_block ==
  note: d_vd_bus_6 in case14gfl
      | $1302.18631108196\,\mathrm{id}_{\mathrm{bus},6}+376.991118430775\,\mathrm{vq}_{\mathrm{bus},6}$
      | Automatically generated on 2025-10-09 21:38:30 .
  Alge_id_bus_6_e431e : Inport
  State_vq_bus_6_681db : Inport  Port=2
  Add_45f75 : Sum
  Constant_1302.18631108196_58a93 : Constant  Value=1302.18631108196
  Constant_376.991118430775_e434a : Constant  Value=376.991118430775
  Product_72558 : Product
  Product_d1184 : Product
  Blockout_d_vd_bus_6_b094f : Outport
  wires:
  Constant_1302.18631108196_58a93/1 -> Product_72558/1
  Alge_id_bus_6_e431e/1 -> Product_72558/2
  Product_d1184/1 -> Add_45f75/2
  Constant_376.991118430775_e434a/1 -> Product_d1184/1
  State_vq_bus_6_681db/1 -> Product_d1184/2
  Product_72558/1 -> Add_45f75/1
  Add_45f75/1 -> Blockout_d_vd_bus_6_b094f/1

== system IEEE14_case/AC_1/d_vd_bus_7_block ==
  note: d_vd_bus_7 in case14gfl
      | $3504.63555759756\,\mathrm{id}_{\mathrm{bus},7}+376.991118430775\,\mathrm{vq}_{\mathrm{bus},7}$
      | Automatically generated on 2025-10-09 21:38:31 .
  Alge_id_bus_7_a7561 : Inport
  State_vq_bus_7_3c6fe : Inport  Port=2
  Add_4dc3a : Sum
  Constant_3504.63555759756_8bb38 : Constant  Value=3504.63555759756
  Constant_376.991118430775_26820 : Constant  Value=376.991118430775
  Product_37962 : Product
  Product_40e3b : Product
  Blockout_d_vd_bus_7_1c15c : Outport
  wires:
  Add_4dc3a/1 -> Blockout_d_vd_bus_7_1c15c/1
  Constant_3504.63555759756_8bb38/1 -> Product_40e3b/1
  Alge_id_bus_7_a7561/1 -> Product_40e3b/2
  Product_37962/1 -> Add_4dc3a/2
  Constant_376.991118430775_26820/1 -> Product_37962/1
  Product_40e3b/1 -> Add_4dc3a/1
  State_vq_bus_7_3c6fe/1 -> Product_37962/2

== system IEEE14_case/AC_1/d_vd_bus_8_block ==
  note: d_vd_bus_8 in case14gfl
      | $2490.79058651093\,\mathrm{id}_{\mathrm{bus},8}+376.991118430775\,\mathrm{vq}_{\mathrm{bus},8}$
      | Automatically generated on 2025-10-09 21:38:33 .
  Alge_id_bus_8_67a63 : Inport
  State_vq_bus_8_e0284 : Inport  Port=2
  Add_4e006 : Sum
  Constant_2490.79058651093_a4825 : Constant  Value=2490.79058651093
  Constant_376.991118430775_b8c33 : Constant  Value=376.991118430775
  Product_ddb59 : Product
  Product_f0ada : Product
  Blockout_d_vd_bus_8_50ae4 : Outport
  wires:
  Add_4e006/1 -> Blockout_d_vd_bus_8_50ae4/1
  Constant_2490.79058651093_a4825/1 -> Product_f0ada/1
  Alge_id_bus_8_67a63/1 -> Product_f0ada/2
  Constant_376.991118430775_b8c33/1 -> Product_ddb59/1
  Product_f0ada/1 -> Add_4e006/1
  State_vq_bus_8_e0284/1 -> Product_ddb59/2
  Product_ddb59/1 -> Add_4e006/2

== system IEEE14_case/AC_1/d_vd_bus_9_block ==
  note: d_vd_bus_9 in case14gfl
      | $1523.0703691556\,\mathrm{id}_{\mathrm{bus},9}+376.991118430775\,\mathrm{vq}_{\mathrm{bus},9}$
      | Automatically generated on 2025-10-09 21:38:34 .
  Alge_id_bus_9_e9a9d : Inport
  State_vq_bus_9_42a9a : Inport  Port=2
  Add_92a2f : Sum
  Constant_1523.0703691556_ad77f : Constant  Value=1523.0703691556
  Constant_376.991118430775_72064 : Constant  Value=376.991118430775
  Product_bde6d : Product
  Product_db397 : Product
  Blockout_d_vd_bus_9_6a7a4 : Outport
  wires:
  Constant_1523.0703691556_ad77f/1 -> Product_db397/1
  Alge_id_bus_9_e9a9d/1 -> Product_db397/2
  Product_bde6d/1 -> Add_92a2f/2
  State_vq_bus_9_42a9a/1 -> Product_bde6d/2
  Constant_376.991118430775_72064/1 -> Product_bde6d/1
  Product_db397/1 -> Add_92a2f/1
  Add_92a2f/1 -> Blockout_d_vd_bus_9_6a7a4/1

== system IEEE14_case/AC_1/d_vq_bus_10_block ==
  note: d_vq_bus_10 in case14gfl
      | $1749.67102824962\,\mathrm{iq}_{\mathrm{bus},10}-376.991118430775\,\mathrm{vd}_{\mathrm{bus},10}$
      | Automatically generated on 2025-10-09 21:38:37 .
  Alge_iq_bus_10_83323 : Inport
  State_vd_bus_10_4ea61 : Inport  Port=2
  Constant_1749.67102824962_2aa2d : Constant  Value=1749.67102824962
  Constant_376.991118430775_3b8af : Constant  Value=376.991118430775
  Product_59f24 : Product
  Product_e0c6c : Product
  Subtract_b8116 : Sum  Inputs=+-
  Blockout_d_vq_bus_10_bbdbe : Outport
  wires:
  Constant_1749.67102824962_2aa2d/1 -> Product_e0c6c/1
  Product_59f24/1 -> Subtract_b8116/2
  Constant_376.991118430775_3b8af/1 -> Product_59f24/1
  Alge_iq_bus_10_83323/1 -> Product_e0c6c/2
  State_vd_bus_10_4ea61/1 -> Product_59f24/2
  Product_e0c6c/1 -> Subtract_b8116/1
  Subtract_b8116/1 -> Blockout_d_vq_bus_10_bbdbe/1
